simulink model "NPC_MPC_rtiFPGASeparationFile"  (R2018b)
settings: Solver=FixedStepAuto  StartTime=0.0  StopTime=Inf  FixedStep=10e-6  RelTol=1e-3
PostLoadFcn:
  | , if any(exist('dsrtsu_mdlpostloadfcn', 'file') ~= 0), dsrtsu_mdlpostloadfcn('Execute', bdroot); end,
values from neighbouring files (symbols this model uses):
  Amplitude = 1    [params.m]
  L = 10e-3    (= 0.01)    [params.m]
  R = 7.5    [params.m]
  S = [-1 -1 -1 ... (first row only)    [params.m]
undefined symbols (not defined in the file or in its folder): T
libraries: xbsIndex_r4 x282, rti1202lib_adc_class1 x3, rtiproclib x3, simulink x1, rtifpgainterfacelib x1
(part 4 of 6)

== system NPC_MPC_rtiFPGASeparationFile/RTI Data ==
  RTI Data Store : Subsystem  Tag="struct('private',struct('version',struct('dsVer',uint32(2),'dsVerCreation',uint32(2),'RTI',struct('ver','7.13','type','RTI1202')),'access',struct('type','Model','isPerm',1,'created',['24-Mar-2026 14:27:03'],'modified',['24-Mar-2026 17:04:08'],'location','')),'public',struct('main',struct('data',[]),'sub',struct('name',{{'NPC_MPC'}},'data',{{struct('TH',struct('thTaskInfo',struct('taskType',{'TIMER','HWINT','TMRINT','SWINT','GLINT'},'tasksNumOf',{1,1,0,0,0},'srcIds',{{'TIMERA'},{'FPGACL1FPGA_INTP0Ch0'},{},{},{}},'taskNames',{{['Timer Task 1']},{'PROC_INT_BL1'},{},{},{}})),'th_tc',struct('dataType',{'TASK','TASK'},'taskGroupId',{'',''},'taskGroupList',{{},{}},'taskSchedulingPolicy',{'FCFS','FCFS'},'taskType',{'TIMER','HWINT'},'blkh',{-1,['NPC_MPC/PROC_INT_BL1/Common Hardware' char(10) 'Interrupt Interface']},'srcId',{'TIMERA','FPGACL1FPGA_INTP0Ch0'},'srcSgnName',{['Timer A interrupt'],['FPGA Type CL1 FPGA_INT Port 0 Channel 0']},'srcCpuName',{'',''},'taskName',{['Timer Task 1  [1e-05] s'],'PROC_INT_BL1'},'taskNameDisplayExt',{'',''},'smplTime',{1e-5,0},'smplTimeOffs',{0,0},'hasFixedPriority',{0,0},'priority',{1,2},'hasFixedOvc',{0,0},'ovcType',{1,1},'ovcMax',{1,1}),'tc_th',struct('dataType',{'TASK','TASK'},'taskGroupId',{'',''},'taskGroupList',{{},{}},'taskSchedulingPolicy',{'FCFS','FCFS'},'taskType',{'TIMER','HWINT'},'blkh',{-1,['NPC_MPC/PROC_INT_BL1/Common Hardware' char(10) 'Interrupt Interface']},'srcId',{'TIMERA','FPGACL1FPGA_INTP0Ch0'},'srcSgnName',{['Timer A interrupt'],['FPGA Type CL1 FPGA_INT Port 0 Channel 0']},'srcCpuName',{'',''},'taskName',{['Timer Task 1  [1e-05] s'],'PROC_INT_BL1'},'taskNameDisplayExt',{'',''},'smplTime',{1e-5,0},'smplTimeOffs',{0,0},'hasFixedPriority',{0,0},'priority',{1,2},'hasFixedOvc',{0,0},'ovcType',{1,1},'ovcMax',{1,1}))}})))"  mask(RTI_DATA_STORE){}
      mask help:
      | RTI Data Store Block. This block is used by RTI to store internal model dependent data. Deleting this block will result in data loss.
      |
      | NEVER DELETE, COPY, OR MODIFY THIS BLOCK!
      mask Help:
      | RTI Data Store Block. This block is used by RTI to store internal model dependent data. Deleting this block will result in data loss.
      | 
      | NEVER DELETE, COPY, OR MODIFY THIS BLOCK!
      mask Display: text(0.5, 0.5, ' ', 'HorizontalAlignment', 'center');

== system NPC_MPC_rtiFPGASeparationFile/Subsystem ==
  iref : Inport
  i : Inport  Port=2
  Trigger : TriggerPort  TriggerType=function-call  VariantControl=Variant  PortDimensions=1
  Constant : Constant  Value=100
  MATLAB Function : MATLAB Function  TreatAsAtomicUnit=on
  Out1 : Outport
  wires:
  i/1 -> MATLAB Function/2(i)
  MATLAB Function/1(state) -> Out1/1
  iref/1 -> MATLAB Function/1(iref)
  Constant/1 -> MATLAB Function/3(Vdc)

== system NPC_MPC_rtiFPGASeparationFile/FPGA/FPGA_INT_BL1 ==
  Int : Inport
  CEP1 : xbsIndex_r4/Clock Enable Probe  inherit_constraints=off  block_type=ceprobe
      settings: infoedit="Clock enable extractor.  Produces a Boolean output that mirrors the hardware clock enable associated with the input sample rate.<br><br>Hardware notes: in hardware this block costs nothing."
  Constant1 : xbsIndex_r4/Constant  const=1  gui_display_data_type=Fixed-point  arith_type=Boolean  n_bits=16  bin_pt=14  preci_type=Single  exp_width=8  frac_width=24  explicit_period=on  period=1*1e-08  equ=P=C  opselect=C  inp2=PCIN>>17  opr=+  inp1=P  carry=CIN  dbl_ovrd=off  block_type=constant
  Convert1 : xbsIndex_r4/Convert  gui_display_data_type=Fixed-point  arith_type=Unsigned  n_bits=1  bin_pt=0  float_type=Single  exp_bits=8  fraction_bits=24  quantization=Truncate  overflow=Wrap  en=off  latency=0  pipeline=off  dbl_ovrd=off  block_type=convert
  Register1 : xbsIndex_r4/Register  init=0  rst=off  en=on  dbl_ovrd=off  block_type=register
  Terminator : Terminator
  phs_interrupt : Subsystem
  usr_interrupt_00 : xbsIndex_r4/Gateway Out  inherit_from_input=off  hdl_port=on  rows=1  columns=1  UseAsDAC=off  DACChannel='1'  interface=None  automatic_assignment=on  address_offset=hex2dec('00')  intf_name=''  intf_description=''  timing_constraint=None  locs_specified=off  LOCs={}  io_standard={}  block_type=gatewayout
  tag scope: CN_NPC_MPC_1_read_Interrupt_1_data_o=global
  wires:
  phs_interrupt/1(data_o) -> [CN_NPC_MPC_1_read_Interrupt_1_data_o], Terminator/1
  usr_interrupt_00/1 -> phs_interrupt/1(data_i)
  Convert1/1 -> Register1/1
  Int/1 -> Convert1/1
  Register1/1 -> usr_interrupt_00/1
  CEP1/1 -> Register1/2
  Constant1/1 -> CEP1/1

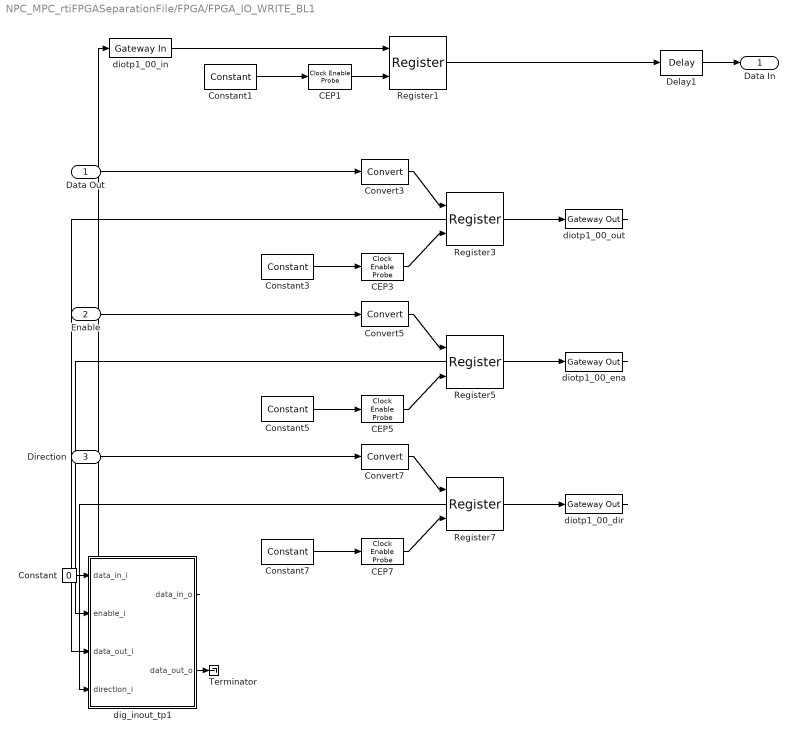
== system NPC_MPC_rtiFPGASeparationFile/FPGA/FPGA_IO_WRITE_BL1 ==
  Data Out : Inport
  Enable : Inport  Port=2
  Direction : Inport  Port=3
  CEP{1,3,5,7} (4 alike) : xbsIndex_r4/Clock Enable Probe  inherit_constraints=off  block_type=ceprobe
      settings: infoedit="Clock enable extractor.  Produces a Boolean output that mirrors the hardware clock enable associated with the input sample rate.<br><br>Hardware notes: in hardware this block costs nothing."
  Constant : Constant  Value=0
  Constant{1,3,5,7} (4 alike) : xbsIndex_r4/Constant  const=1  gui_display_data_type=Fixed-point  arith_type=Boolean  n_bits=16  bin_pt=14  preci_type=Single  exp_width=8  frac_width=24  explicit_period=on  period=1*1e-08  equ=P=C  opselect=C  inp2=PCIN>>17  opr=+  inp1=P  carry=CIN  dbl_ovrd=off  block_type=constant
  Convert3 : xbsIndex_r4/Convert  gui_display_data_type=Fixed-point  arith_type=Unsigned  n_bits=1  bin_pt=0  float_type=Single  exp_bits=8  fraction_bits=24  quantization=Truncate  overflow=Wrap  en=off  latency=0  pipeline=off  dbl_ovrd=off  block_type=convert
  Convert5 : xbsIndex_r4/Convert  gui_display_data_type=Fixed-point  arith_type=Unsigned  n_bits=1  bin_pt=0  float_type=Single  exp_bits=8  fraction_bits=24  quantization=Truncate  overflow=Wrap  en=off  latency=0  pipeline=off  dbl_ovrd=off  block_type=convert
  Convert7 : xbsIndex_r4/Convert  gui_display_data_type=Fixed-point  arith_type=Unsigned  n_bits=1  bin_pt=0  float_type=Single  exp_bits=8  fraction_bits=24  quantization=Truncate  overflow=Wrap  en=off  latency=0  pipeline=off  dbl_ovrd=off  block_type=convert
  Delay1 : xbsIndex_r4/Delay  rst=off  infoeditControl=Selection of Reset will increase slice count due to use of real FFs and instead of SRLs  en=off  latency=0  reg_retiming=off  dbl_ovrd=off  block_type=delay
  Register{1,3,5,7} (4 alike) : xbsIndex_r4/Register  init=0  rst=off  en=on  dbl_ovrd=off  block_type=register
  Terminator : Terminator
  dig_inout_tp1 : Subsystem
      mask init:
      | par = rtifpgafcnlib('GetCurrentParaValue', get_param(get(gcbh, 'parent'), 'handle'));
      | inverted_dio = str2double(par(2).Value{1});
      | vsetting = str2double(par(5).Value{1});
      | switch vsetting 
      |     case 1
      |         voltage = 3.3
      |     case 2
      |         voltage = 2.5;
      |     otherwise
      |         voltage = 5;
      | end
  diotp1_00_dir : xbsIndex_r4/Gateway Out  inherit_from_input=off  hdl_port=on  rows=1  columns=1  UseAsDAC=off  DACChannel='1'  interface=None  automatic_assignment=on  address_offset=hex2dec('00')  intf_name=''  intf_description=''  timing_constraint=None  locs_specified=off  LOCs={}  io_standard={}  block_type=gatewayout
  diotp1_00_ena : xbsIndex_r4/Gateway Out  inherit_from_input=off  hdl_port=on  rows=1  columns=1  UseAsDAC=off  DACChannel='1'  interface=None  automatic_assignment=on  address_offset=hex2dec('00')  intf_name=''  intf_description=''  timing_constraint=None  locs_specified=off  LOCs={}  io_standard={}  block_type=gatewayout
  diotp1_00_in : xbsIndex_r4/Gateway In  gui_display_data_type=Fixed-point  arith_type=Unsigned  n_bits=1  bin_pt=0  preci_type=Single  exp_width=8  frac_width=24  rows=1  columns=1  quantization="Round  (unbiased: +/- Inf)"  overflow=Saturate  period=1e-08  UseAsADC=off  ADCChannel='1'  interface=None  automatic_assignment=on  address_offset=hex2dec('00')  intf_name=''  intf_description=''  default_value=0  timing_constraint=None  locs_specified=off  LOCs={}  io_standard={}  inherit_from_input=off  hdl_port=on  dbl_ovrd=off  block_type=gatewayin
  diotp1_00_out : xbsIndex_r4/Gateway Out  inherit_from_input=off  hdl_port=on  rows=1  columns=1  UseAsDAC=off  DACChannel='1'  interface=None  automatic_assignment=on  address_offset=hex2dec('00')  intf_name=''  intf_description=''  timing_constraint=None  locs_specified=off  LOCs={}  io_standard={}  block_type=gatewayout
  Data In : Outport
  wires:
  dig_inout_tp1/2(data_out_o) -> Terminator/1
  Constant/1 -> dig_inout_tp1/1(data_in_i)
  diotp1_00_dir/1 -> dig_inout_tp1/4(direction_i)
  diotp1_00_ena/1 -> dig_inout_tp1/2(enable_i)
  diotp1_00_out/1 -> dig_inout_tp1/3(data_out_i)
  dig_inout_tp1/1(data_in_o) -> diotp1_00_in/1
  Convert7/1 -> Register7/1
  Direction/1 -> Convert7/1
  Register7/1 -> diotp1_00_dir/1
  CEP7/1 -> Register7/2
  Constant7/1 -> CEP7/1
  Convert5/1 -> Register5/1
  Enable/1 -> Convert5/1
  Register5/1 -> diotp1_00_ena/1
  CEP5/1 -> Register5/2
  Constant5/1 -> CEP5/1
  Convert3/1 -> Register3/1
  Data Out/1 -> Convert3/1
  Register3/1 -> diotp1_00_out/1
  CEP3/1 -> Register3/2
  Constant3/1 -> CEP3/1
  diotp1_00_in/1 -> Register1/1
  CEP1/1 -> Register1/2
  Constant1/1 -> CEP1/1
  Delay1/1 -> Data In/1
  Register1/1 -> Delay1/1

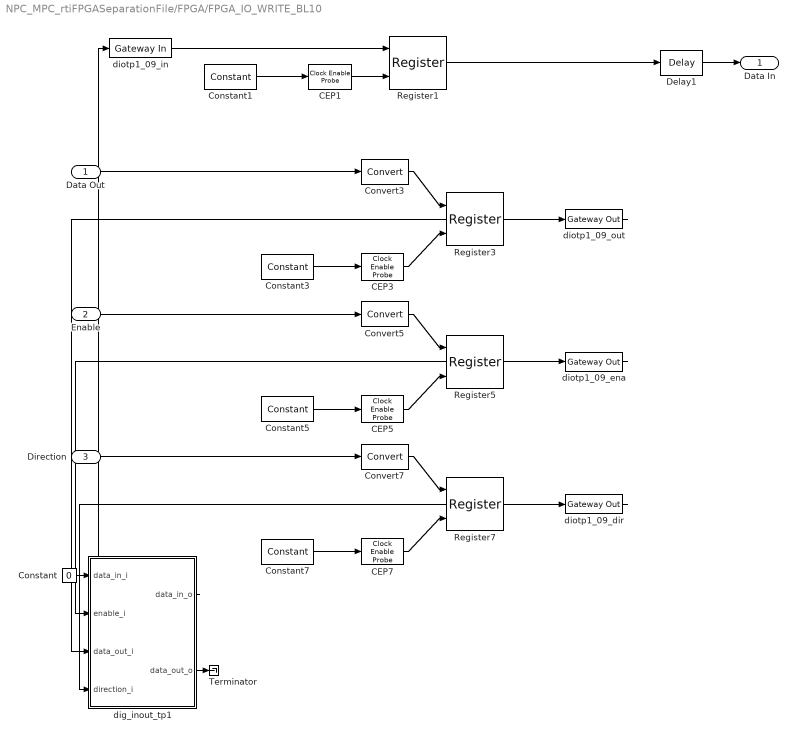
== system NPC_MPC_rtiFPGASeparationFile/FPGA/FPGA_IO_WRITE_BL10 ==
  Data Out : Inport
  Enable : Inport  Port=2
  Direction : Inport  Port=3
  CEP{1,3,5,7} (4 alike) : xbsIndex_r4/Clock Enable Probe  inherit_constraints=off  block_type=ceprobe
      settings: infoedit="Clock enable extractor.  Produces a Boolean output that mirrors the hardware clock enable associated with the input sample rate.<br><br>Hardware notes: in hardware this block costs nothing."
  Constant : Constant  Value=0
  Constant{1,3,5,7} (4 alike) : xbsIndex_r4/Constant  const=1  gui_display_data_type=Fixed-point  arith_type=Boolean  n_bits=16  bin_pt=14  preci_type=Single  exp_width=8  frac_width=24  explicit_period=on  period=1*1e-08  equ=P=C  opselect=C  inp2=PCIN>>17  opr=+  inp1=P  carry=CIN  dbl_ovrd=off  block_type=constant
  Convert3 : xbsIndex_r4/Convert  gui_display_data_type=Fixed-point  arith_type=Unsigned  n_bits=1  bin_pt=0  float_type=Single  exp_bits=8  fraction_bits=24  quantization=Truncate  overflow=Wrap  en=off  latency=0  pipeline=off  dbl_ovrd=off  block_type=convert
  Convert5 : xbsIndex_r4/Convert  gui_display_data_type=Fixed-point  arith_type=Unsigned  n_bits=1  bin_pt=0  float_type=Single  exp_bits=8  fraction_bits=24  quantization=Truncate  overflow=Wrap  en=off  latency=0  pipeline=off  dbl_ovrd=off  block_type=convert
  Convert7 : xbsIndex_r4/Convert  gui_display_data_type=Fixed-point  arith_type=Unsigned  n_bits=1  bin_pt=0  float_type=Single  exp_bits=8  fraction_bits=24  quantization=Truncate  overflow=Wrap  en=off  latency=0  pipeline=off  dbl_ovrd=off  block_type=convert
  Delay1 : xbsIndex_r4/Delay  rst=off  infoeditControl=Selection of Reset will increase slice count due to use of real FFs and instead of SRLs  en=off  latency=0  reg_retiming=off  dbl_ovrd=off  block_type=delay
  Register{1,3,5,7} (4 alike) : xbsIndex_r4/Register  init=0  rst=off  en=on  dbl_ovrd=off  block_type=register
  Terminator : Terminator
  dig_inout_tp1 : Subsystem
      mask init: same as NPC_MPC_rtiFPGASeparationFile/FPGA/FPGA_IO_WRITE_BL1/dig_inout_tp1
  diotp1_09_dir : xbsIndex_r4/Gateway Out  inherit_from_input=off  hdl_port=on  rows=1  columns=1  UseAsDAC=off  DACChannel='1'  interface=None  automatic_assignment=on  address_offset=hex2dec('00')  intf_name=''  intf_description=''  timing_constraint=None  locs_specified=off  LOCs={}  io_standard={}  block_type=gatewayout
  diotp1_09_ena : xbsIndex_r4/Gateway Out  inherit_from_input=off  hdl_port=on  rows=1  columns=1  UseAsDAC=off  DACChannel='1'  interface=None  automatic_assignment=on  address_offset=hex2dec('00')  intf_name=''  intf_description=''  timing_constraint=None  locs_specified=off  LOCs={}  io_standard={}  block_type=gatewayout
  diotp1_09_in : xbsIndex_r4/Gateway In  gui_display_data_type=Fixed-point  arith_type=Unsigned  n_bits=1  bin_pt=0  preci_type=Single  exp_width=8  frac_width=24  rows=1  columns=1  quantization="Round  (unbiased: +/- Inf)"  overflow=Saturate  period=1e-08  UseAsADC=off  ADCChannel='1'  interface=None  automatic_assignment=on  address_offset=hex2dec('00')  intf_name=''  intf_description=''  default_value=0  timing_constraint=None  locs_specified=off  LOCs={}  io_standard={}  inherit_from_input=off  hdl_port=on  dbl_ovrd=off  block_type=gatewayin
  diotp1_09_out : xbsIndex_r4/Gateway Out  inherit_from_input=off  hdl_port=on  rows=1  columns=1  UseAsDAC=off  DACChannel='1'  interface=None  automatic_assignment=on  address_offset=hex2dec('00')  intf_name=''  intf_description=''  timing_constraint=None  locs_specified=off  LOCs={}  io_standard={}  block_type=gatewayout
  Data In : Outport
  wires:
  dig_inout_tp1/2(data_out_o) -> Terminator/1
  Constant/1 -> dig_inout_tp1/1(data_in_i)
  diotp1_09_dir/1 -> dig_inout_tp1/4(direction_i)
  diotp1_09_ena/1 -> dig_inout_tp1/2(enable_i)
  diotp1_09_out/1 -> dig_inout_tp1/3(data_out_i)
  dig_inout_tp1/1(data_in_o) -> diotp1_09_in/1
  Convert7/1 -> Register7/1
  Direction/1 -> Convert7/1
  Register7/1 -> diotp1_09_dir/1
  CEP7/1 -> Register7/2
  Constant7/1 -> CEP7/1
  Convert5/1 -> Register5/1
  Enable/1 -> Convert5/1
  Register5/1 -> diotp1_09_ena/1
  CEP5/1 -> Register5/2
  Constant5/1 -> CEP5/1
  Convert3/1 -> Register3/1
  Data Out/1 -> Convert3/1
  Register3/1 -> diotp1_09_out/1
  CEP3/1 -> Register3/2
  Constant3/1 -> CEP3/1
  diotp1_09_in/1 -> Register1/1
  CEP1/1 -> Register1/2
  Constant1/1 -> CEP1/1
  Delay1/1 -> Data In/1
  Register1/1 -> Delay1/1

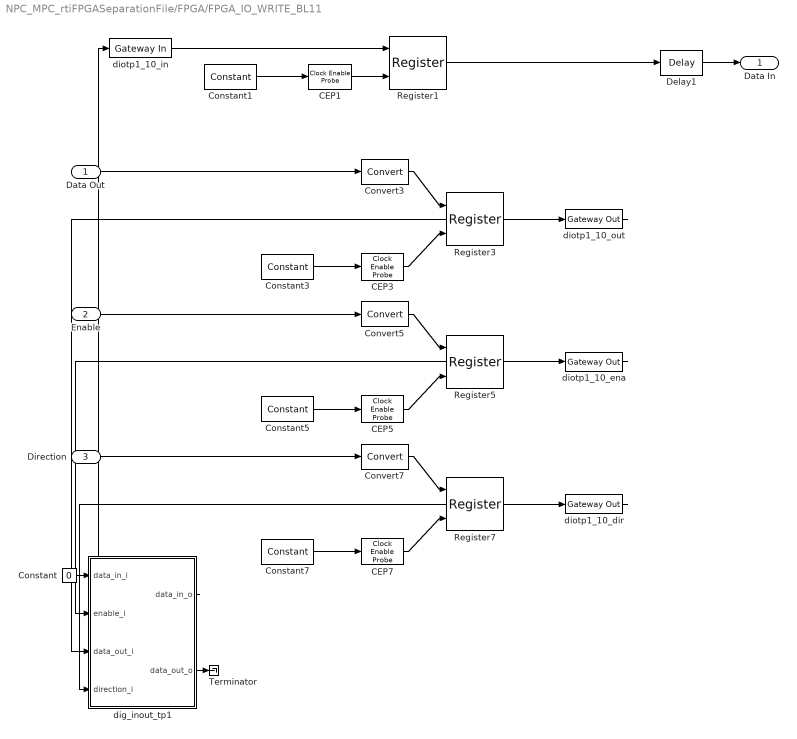
== system NPC_MPC_rtiFPGASeparationFile/FPGA/FPGA_IO_WRITE_BL11 ==
  Data Out : Inport
  Enable : Inport  Port=2
  Direction : Inport  Port=3
  CEP{1,3,5,7} (4 alike) : xbsIndex_r4/Clock Enable Probe  inherit_constraints=off  block_type=ceprobe
      settings: infoedit="Clock enable extractor.  Produces a Boolean output that mirrors the hardware clock enable associated with the input sample rate.<br><br>Hardware notes: in hardware this block costs nothing."
  Constant : Constant  Value=0
  Constant{1,3,5,7} (4 alike) : xbsIndex_r4/Constant  const=1  gui_display_data_type=Fixed-point  arith_type=Boolean  n_bits=16  bin_pt=14  preci_type=Single  exp_width=8  frac_width=24  explicit_period=on  period=1*1e-08  equ=P=C  opselect=C  inp2=PCIN>>17  opr=+  inp1=P  carry=CIN  dbl_ovrd=off  block_type=constant
  Convert3 : xbsIndex_r4/Convert  gui_display_data_type=Fixed-point  arith_type=Unsigned  n_bits=1  bin_pt=0  float_type=Single  exp_bits=8  fraction_bits=24  quantization=Truncate  overflow=Wrap  en=off  latency=0  pipeline=off  dbl_ovrd=off  block_type=convert
  Convert5 : xbsIndex_r4/Convert  gui_display_data_type=Fixed-point  arith_type=Unsigned  n_bits=1  bin_pt=0  float_type=Single  exp_bits=8  fraction_bits=24  quantization=Truncate  overflow=Wrap  en=off  latency=0  pipeline=off  dbl_ovrd=off  block_type=convert
  Convert7 : xbsIndex_r4/Convert  gui_display_data_type=Fixed-point  arith_type=Unsigned  n_bits=1  bin_pt=0  float_type=Single  exp_bits=8  fraction_bits=24  quantization=Truncate  overflow=Wrap  en=off  latency=0  pipeline=off  dbl_ovrd=off  block_type=convert
  Delay1 : xbsIndex_r4/Delay  rst=off  infoeditControl=Selection of Reset will increase slice count due to use of real FFs and instead of SRLs  en=off  latency=0  reg_retiming=off  dbl_ovrd=off  block_type=delay
  Register{1,3,5,7} (4 alike) : xbsIndex_r4/Register  init=0  rst=off  en=on  dbl_ovrd=off  block_type=register
  Terminator : Terminator
  dig_inout_tp1 : Subsystem
      mask init: same as NPC_MPC_rtiFPGASeparationFile/FPGA/FPGA_IO_WRITE_BL1/dig_inout_tp1
  diotp1_10_dir : xbsIndex_r4/Gateway Out  inherit_from_input=off  hdl_port=on  rows=1  columns=1  UseAsDAC=off  DACChannel='1'  interface=None  automatic_assignment=on  address_offset=hex2dec('00')  intf_name=''  intf_description=''  timing_constraint=None  locs_specified=off  LOCs={}  io_standard={}  block_type=gatewayout
  diotp1_10_ena : xbsIndex_r4/Gateway Out  inherit_from_input=off  hdl_port=on  rows=1  columns=1  UseAsDAC=off  DACChannel='1'  interface=None  automatic_assignment=on  address_offset=hex2dec('00')  intf_name=''  intf_description=''  timing_constraint=None  locs_specified=off  LOCs={}  io_standard={}  block_type=gatewayout
  diotp1_10_in : xbsIndex_r4/Gateway In  gui_display_data_type=Fixed-point  arith_type=Unsigned  n_bits=1  bin_pt=0  preci_type=Single  exp_width=8  frac_width=24  rows=1  columns=1  quantization="Round  (unbiased: +/- Inf)"  overflow=Saturate  period=1e-08  UseAsADC=off  ADCChannel='1'  interface=None  automatic_assignment=on  address_offset=hex2dec('00')  intf_name=''  intf_description=''  default_value=0  timing_constraint=None  locs_specified=off  LOCs={}  io_standard={}  inherit_from_input=off  hdl_port=on  dbl_ovrd=off  block_type=gatewayin
  diotp1_10_out : xbsIndex_r4/Gateway Out  inherit_from_input=off  hdl_port=on  rows=1  columns=1  UseAsDAC=off  DACChannel='1'  interface=None  automatic_assignment=on  address_offset=hex2dec('00')  intf_name=''  intf_description=''  timing_constraint=None  locs_specified=off  LOCs={}  io_standard={}  block_type=gatewayout
  Data In : Outport
  wires:
  dig_inout_tp1/2(data_out_o) -> Terminator/1
  Constant/1 -> dig_inout_tp1/1(data_in_i)
  diotp1_10_dir/1 -> dig_inout_tp1/4(direction_i)
  diotp1_10_ena/1 -> dig_inout_tp1/2(enable_i)
  diotp1_10_out/1 -> dig_inout_tp1/3(data_out_i)
  dig_inout_tp1/1(data_in_o) -> diotp1_10_in/1
  Convert7/1 -> Register7/1
  Direction/1 -> Convert7/1
  Register7/1 -> diotp1_10_dir/1
  CEP7/1 -> Register7/2
  Constant7/1 -> CEP7/1
  Convert5/1 -> Register5/1
  Enable/1 -> Convert5/1
  Register5/1 -> diotp1_10_ena/1
  CEP5/1 -> Register5/2
  Constant5/1 -> CEP5/1
  Convert3/1 -> Register3/1
  Data Out/1 -> Convert3/1
  Register3/1 -> diotp1_10_out/1
  CEP3/1 -> Register3/2
  Constant3/1 -> CEP3/1
  diotp1_10_in/1 -> Register1/1
  CEP1/1 -> Register1/2
  Constant1/1 -> CEP1/1
  Delay1/1 -> Data In/1
  Register1/1 -> Delay1/1

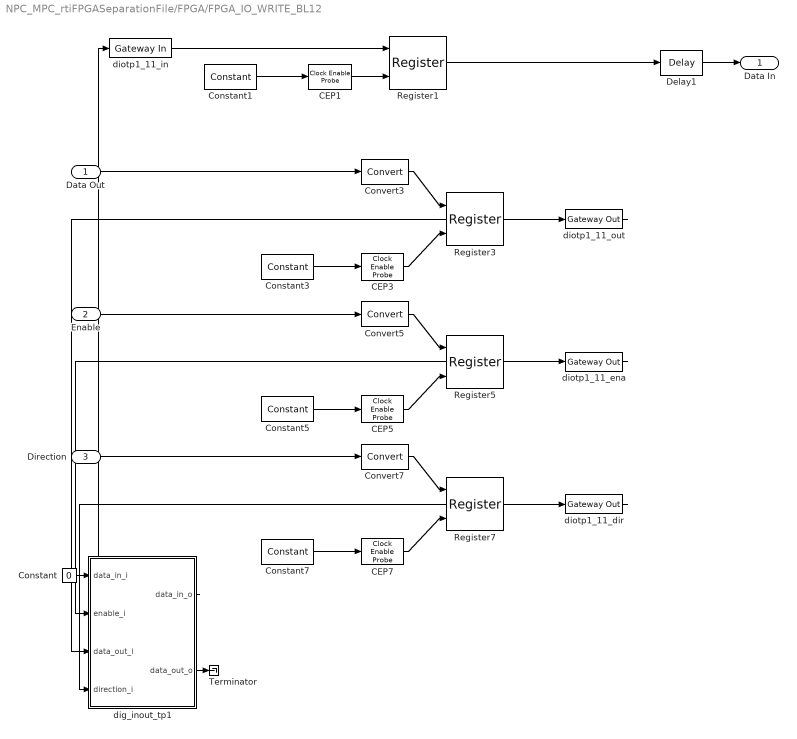
== system NPC_MPC_rtiFPGASeparationFile/FPGA/FPGA_IO_WRITE_BL12 ==
  Data Out : Inport
  Enable : Inport  Port=2
  Direction : Inport  Port=3
  CEP{1,3,5,7} (4 alike) : xbsIndex_r4/Clock Enable Probe  inherit_constraints=off  block_type=ceprobe
      settings: infoedit="Clock enable extractor.  Produces a Boolean output that mirrors the hardware clock enable associated with the input sample rate.<br><br>Hardware notes: in hardware this block costs nothing."
  Constant : Constant  Value=0
  Constant{1,3,5,7} (4 alike) : xbsIndex_r4/Constant  const=1  gui_display_data_type=Fixed-point  arith_type=Boolean  n_bits=16  bin_pt=14  preci_type=Single  exp_width=8  frac_width=24  explicit_period=on  period=1*1e-08  equ=P=C  opselect=C  inp2=PCIN>>17  opr=+  inp1=P  carry=CIN  dbl_ovrd=off  block_type=constant
  Convert3 : xbsIndex_r4/Convert  gui_display_data_type=Fixed-point  arith_type=Unsigned  n_bits=1  bin_pt=0  float_type=Single  exp_bits=8  fraction_bits=24  quantization=Truncate  overflow=Wrap  en=off  latency=0  pipeline=off  dbl_ovrd=off  block_type=convert
  Convert5 : xbsIndex_r4/Convert  gui_display_data_type=Fixed-point  arith_type=Unsigned  n_bits=1  bin_pt=0  float_type=Single  exp_bits=8  fraction_bits=24  quantization=Truncate  overflow=Wrap  en=off  latency=0  pipeline=off  dbl_ovrd=off  block_type=convert
  Convert7 : xbsIndex_r4/Convert  gui_display_data_type=Fixed-point  arith_type=Unsigned  n_bits=1  bin_pt=0  float_type=Single  exp_bits=8  fraction_bits=24  quantization=Truncate  overflow=Wrap  en=off  latency=0  pipeline=off  dbl_ovrd=off  block_type=convert
  Delay1 : xbsIndex_r4/Delay  rst=off  infoeditControl=Selection of Reset will increase slice count due to use of real FFs and instead of SRLs  en=off  latency=0  reg_retiming=off  dbl_ovrd=off  block_type=delay
  Register{1,3,5,7} (4 alike) : xbsIndex_r4/Register  init=0  rst=off  en=on  dbl_ovrd=off  block_type=register
  Terminator : Terminator
  dig_inout_tp1 : Subsystem
      mask init: same as NPC_MPC_rtiFPGASeparationFile/FPGA/FPGA_IO_WRITE_BL1/dig_inout_tp1
  diotp1_11_dir : xbsIndex_r4/Gateway Out  inherit_from_input=off  hdl_port=on  rows=1  columns=1  UseAsDAC=off  DACChannel='1'  interface=None  automatic_assignment=on  address_offset=hex2dec('00')  intf_name=''  intf_description=''  timing_constraint=None  locs_specified=off  LOCs={}  io_standard={}  block_type=gatewayout
  diotp1_11_ena : xbsIndex_r4/Gateway Out  inherit_from_input=off  hdl_port=on  rows=1  columns=1  UseAsDAC=off  DACChannel='1'  interface=None  automatic_assignment=on  address_offset=hex2dec('00')  intf_name=''  intf_description=''  timing_constraint=None  locs_specified=off  LOCs={}  io_standard={}  block_type=gatewayout
  diotp1_11_in : xbsIndex_r4/Gateway In  gui_display_data_type=Fixed-point  arith_type=Unsigned  n_bits=1  bin_pt=0  preci_type=Single  exp_width=8  frac_width=24  rows=1  columns=1  quantization="Round  (unbiased: +/- Inf)"  overflow=Saturate  period=1e-08  UseAsADC=off  ADCChannel='1'  interface=None  automatic_assignment=on  address_offset=hex2dec('00')  intf_name=''  intf_description=''  default_value=0  timing_constraint=None  locs_specified=off  LOCs={}  io_standard={}  inherit_from_input=off  hdl_port=on  dbl_ovrd=off  block_type=gatewayin
  diotp1_11_out : xbsIndex_r4/Gateway Out  inherit_from_input=off  hdl_port=on  rows=1  columns=1  UseAsDAC=off  DACChannel='1'  interface=None  automatic_assignment=on  address_offset=hex2dec('00')  intf_name=''  intf_description=''  timing_constraint=None  locs_specified=off  LOCs={}  io_standard={}  block_type=gatewayout
  Data In : Outport
  wires:
  dig_inout_tp1/2(data_out_o) -> Terminator/1
  Constant/1 -> dig_inout_tp1/1(data_in_i)
  diotp1_11_dir/1 -> dig_inout_tp1/4(direction_i)
  diotp1_11_ena/1 -> dig_inout_tp1/2(enable_i)
  diotp1_11_out/1 -> dig_inout_tp1/3(data_out_i)
  dig_inout_tp1/1(data_in_o) -> diotp1_11_in/1
  Convert7/1 -> Register7/1
  Direction/1 -> Convert7/1
  Register7/1 -> diotp1_11_dir/1
  CEP7/1 -> Register7/2
  Constant7/1 -> CEP7/1
  Convert5/1 -> Register5/1
  Enable/1 -> Convert5/1
  Register5/1 -> diotp1_11_ena/1
  CEP5/1 -> Register5/2
  Constant5/1 -> CEP5/1
  Convert3/1 -> Register3/1
  Data Out/1 -> Convert3/1
  Register3/1 -> diotp1_11_out/1
  CEP3/1 -> Register3/2
  Constant3/1 -> CEP3/1
  diotp1_11_in/1 -> Register1/1
  CEP1/1 -> Register1/2
  Constant1/1 -> CEP1/1
  Delay1/1 -> Data In/1
  Register1/1 -> Delay1/1

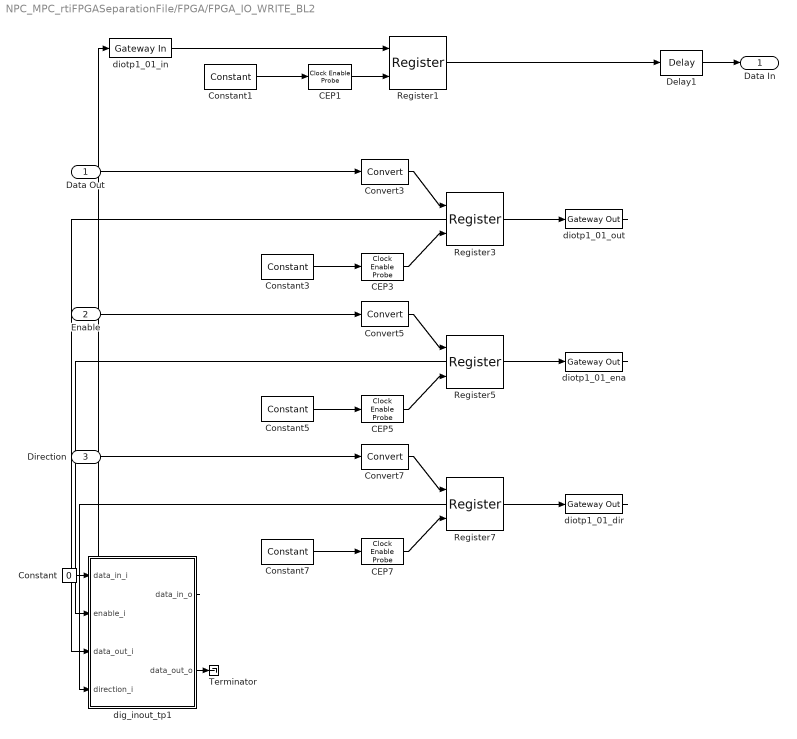
== system NPC_MPC_rtiFPGASeparationFile/FPGA/FPGA_IO_WRITE_BL2 ==
  Data Out : Inport
  Enable : Inport  Port=2
  Direction : Inport  Port=3
  CEP{1,3,5,7} (4 alike) : xbsIndex_r4/Clock Enable Probe  inherit_constraints=off  block_type=ceprobe
      settings: infoedit="Clock enable extractor.  Produces a Boolean output that mirrors the hardware clock enable associated with the input sample rate.<br><br>Hardware notes: in hardware this block costs nothing."
  Constant : Constant  Value=0
  Constant{1,3,5,7} (4 alike) : xbsIndex_r4/Constant  const=1  gui_display_data_type=Fixed-point  arith_type=Boolean  n_bits=16  bin_pt=14  preci_type=Single  exp_width=8  frac_width=24  explicit_period=on  period=1*1e-08  equ=P=C  opselect=C  inp2=PCIN>>17  opr=+  inp1=P  carry=CIN  dbl_ovrd=off  block_type=constant
  Convert3 : xbsIndex_r4/Convert  gui_display_data_type=Fixed-point  arith_type=Unsigned  n_bits=1  bin_pt=0  float_type=Single  exp_bits=8  fraction_bits=24  quantization=Truncate  overflow=Wrap  en=off  latency=0  pipeline=off  dbl_ovrd=off  block_type=convert
  Convert5 : xbsIndex_r4/Convert  gui_display_data_type=Fixed-point  arith_type=Unsigned  n_bits=1  bin_pt=0  float_type=Single  exp_bits=8  fraction_bits=24  quantization=Truncate  overflow=Wrap  en=off  latency=0  pipeline=off  dbl_ovrd=off  block_type=convert
  Convert7 : xbsIndex_r4/Convert  gui_display_data_type=Fixed-point  arith_type=Unsigned  n_bits=1  bin_pt=0  float_type=Single  exp_bits=8  fraction_bits=24  quantization=Truncate  overflow=Wrap  en=off  latency=0  pipeline=off  dbl_ovrd=off  block_type=convert
  Delay1 : xbsIndex_r4/Delay  rst=off  infoeditControl=Selection of Reset will increase slice count due to use of real FFs and instead of SRLs  en=off  latency=0  reg_retiming=off  dbl_ovrd=off  block_type=delay
  Register{1,3,5,7} (4 alike) : xbsIndex_r4/Register  init=0  rst=off  en=on  dbl_ovrd=off  block_type=register
  Terminator : Terminator
  dig_inout_tp1 : Subsystem
      mask init: same as NPC_MPC_rtiFPGASeparationFile/FPGA/FPGA_IO_WRITE_BL1/dig_inout_tp1
  diotp1_01_dir : xbsIndex_r4/Gateway Out  inherit_from_input=off  hdl_port=on  rows=1  columns=1  UseAsDAC=off  DACChannel='1'  interface=None  automatic_assignment=on  address_offset=hex2dec('00')  intf_name=''  intf_description=''  timing_constraint=None  locs_specified=off  LOCs={}  io_standard={}  block_type=gatewayout
  diotp1_01_ena : xbsIndex_r4/Gateway Out  inherit_from_input=off  hdl_port=on  rows=1  columns=1  UseAsDAC=off  DACChannel='1'  interface=None  automatic_assignment=on  address_offset=hex2dec('00')  intf_name=''  intf_description=''  timing_constraint=None  locs_specified=off  LOCs={}  io_standard={}  block_type=gatewayout
  diotp1_01_in : xbsIndex_r4/Gateway In  gui_display_data_type=Fixed-point  arith_type=Unsigned  n_bits=1  bin_pt=0  preci_type=Single  exp_width=8  frac_width=24  rows=1  columns=1  quantization="Round  (unbiased: +/- Inf)"  overflow=Saturate  period=1e-08  UseAsADC=off  ADCChannel='1'  interface=None  automatic_assignment=on  address_offset=hex2dec('00')  intf_name=''  intf_description=''  default_value=0  timing_constraint=None  locs_specified=off  LOCs={}  io_standard={}  inherit_from_input=off  hdl_port=on  dbl_ovrd=off  block_type=gatewayin
  diotp1_01_out : xbsIndex_r4/Gateway Out  inherit_from_input=off  hdl_port=on  rows=1  columns=1  UseAsDAC=off  DACChannel='1'  interface=None  automatic_assignment=on  address_offset=hex2dec('00')  intf_name=''  intf_description=''  timing_constraint=None  locs_specified=off  LOCs={}  io_standard={}  block_type=gatewayout
  Data In : Outport
  wires:
  dig_inout_tp1/2(data_out_o) -> Terminator/1
  Constant/1 -> dig_inout_tp1/1(data_in_i)
  diotp1_01_dir/1 -> dig_inout_tp1/4(direction_i)
  diotp1_01_ena/1 -> dig_inout_tp1/2(enable_i)
  diotp1_01_out/1 -> dig_inout_tp1/3(data_out_i)
  dig_inout_tp1/1(data_in_o) -> diotp1_01_in/1
  Convert7/1 -> Register7/1
  Direction/1 -> Convert7/1
  Register7/1 -> diotp1_01_dir/1
  CEP7/1 -> Register7/2
  Constant7/1 -> CEP7/1
  Convert5/1 -> Register5/1
  Enable/1 -> Convert5/1
  Register5/1 -> diotp1_01_ena/1
  CEP5/1 -> Register5/2
  Constant5/1 -> CEP5/1
  Convert3/1 -> Register3/1
  Data Out/1 -> Convert3/1
  Register3/1 -> diotp1_01_out/1
  CEP3/1 -> Register3/2
  Constant3/1 -> CEP3/1
  diotp1_01_in/1 -> Register1/1
  CEP1/1 -> Register1/2
  Constant1/1 -> CEP1/1
  Delay1/1 -> Data In/1
  Register1/1 -> Delay1/1

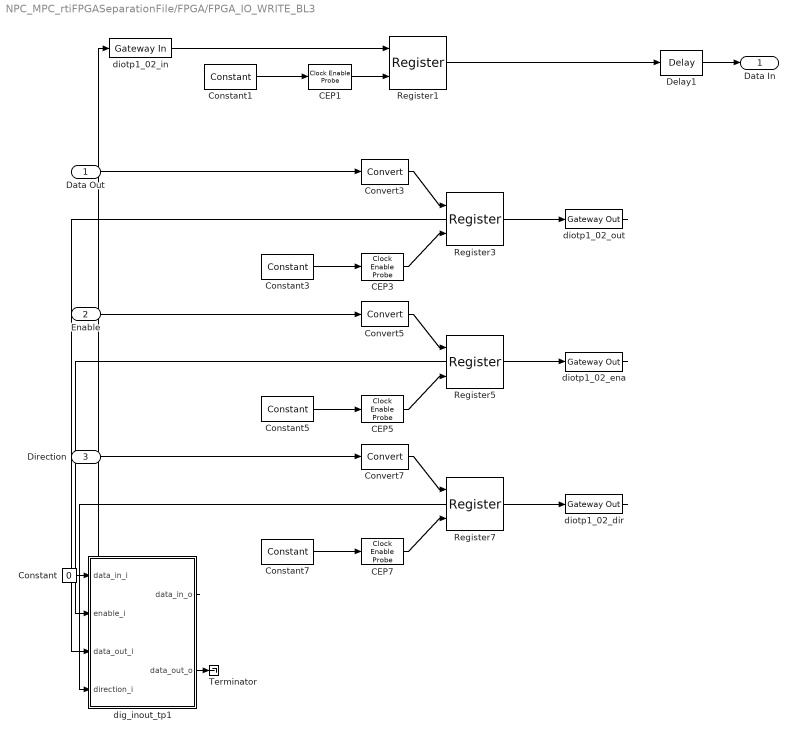
== system NPC_MPC_rtiFPGASeparationFile/FPGA/FPGA_IO_WRITE_BL3 ==
  Data Out : Inport
  Enable : Inport  Port=2
  Direction : Inport  Port=3
  CEP{1,3,5,7} (4 alike) : xbsIndex_r4/Clock Enable Probe  inherit_constraints=off  block_type=ceprobe
      settings: infoedit="Clock enable extractor.  Produces a Boolean output that mirrors the hardware clock enable associated with the input sample rate.<br><br>Hardware notes: in hardware this block costs nothing."
  Constant : Constant  Value=0
  Constant{1,3,5,7} (4 alike) : xbsIndex_r4/Constant  const=1  gui_display_data_type=Fixed-point  arith_type=Boolean  n_bits=16  bin_pt=14  preci_type=Single  exp_width=8  frac_width=24  explicit_period=on  period=1*1e-08  equ=P=C  opselect=C  inp2=PCIN>>17  opr=+  inp1=P  carry=CIN  dbl_ovrd=off  block_type=constant
  Convert3 : xbsIndex_r4/Convert  gui_display_data_type=Fixed-point  arith_type=Unsigned  n_bits=1  bin_pt=0  float_type=Single  exp_bits=8  fraction_bits=24  quantization=Truncate  overflow=Wrap  en=off  latency=0  pipeline=off  dbl_ovrd=off  block_type=convert
  Convert5 : xbsIndex_r4/Convert  gui_display_data_type=Fixed-point  arith_type=Unsigned  n_bits=1  bin_pt=0  float_type=Single  exp_bits=8  fraction_bits=24  quantization=Truncate  overflow=Wrap  en=off  latency=0  pipeline=off  dbl_ovrd=off  block_type=convert
  Convert7 : xbsIndex_r4/Convert  gui_display_data_type=Fixed-point  arith_type=Unsigned  n_bits=1  bin_pt=0  float_type=Single  exp_bits=8  fraction_bits=24  quantization=Truncate  overflow=Wrap  en=off  latency=0  pipeline=off  dbl_ovrd=off  block_type=convert
  Delay1 : xbsIndex_r4/Delay  rst=off  infoeditControl=Selection of Reset will increase slice count due to use of real FFs and instead of SRLs  en=off  latency=0  reg_retiming=off  dbl_ovrd=off  block_type=delay
  Register{1,3,5,7} (4 alike) : xbsIndex_r4/Register  init=0  rst=off  en=on  dbl_ovrd=off  block_type=register
  Terminator : Terminator
  dig_inout_tp1 : Subsystem
      mask init: same as NPC_MPC_rtiFPGASeparationFile/FPGA/FPGA_IO_WRITE_BL1/dig_inout_tp1
  diotp1_02_dir : xbsIndex_r4/Gateway Out  inherit_from_input=off  hdl_port=on  rows=1  columns=1  UseAsDAC=off  DACChannel='1'  interface=None  automatic_assignment=on  address_offset=hex2dec('00')  intf_name=''  intf_description=''  timing_constraint=None  locs_specified=off  LOCs={}  io_standard={}  block_type=gatewayout
  diotp1_02_ena : xbsIndex_r4/Gateway Out  inherit_from_input=off  hdl_port=on  rows=1  columns=1  UseAsDAC=off  DACChannel='1'  interface=None  automatic_assignment=on  address_offset=hex2dec('00')  intf_name=''  intf_description=''  timing_constraint=None  locs_specified=off  LOCs={}  io_standard={}  block_type=gatewayout
  diotp1_02_in : xbsIndex_r4/Gateway In  gui_display_data_type=Fixed-point  arith_type=Unsigned  n_bits=1  bin_pt=0  preci_type=Single  exp_width=8  frac_width=24  rows=1  columns=1  quantization="Round  (unbiased: +/- Inf)"  overflow=Saturate  period=1e-08  UseAsADC=off  ADCChannel='1'  interface=None  automatic_assignment=on  address_offset=hex2dec('00')  intf_name=''  intf_description=''  default_value=0  timing_constraint=None  locs_specified=off  LOCs={}  io_standard={}  inherit_from_input=off  hdl_port=on  dbl_ovrd=off  block_type=gatewayin
  diotp1_02_out : xbsIndex_r4/Gateway Out  inherit_from_input=off  hdl_port=on  rows=1  columns=1  UseAsDAC=off  DACChannel='1'  interface=None  automatic_assignment=on  address_offset=hex2dec('00')  intf_name=''  intf_description=''  timing_constraint=None  locs_specified=off  LOCs={}  io_standard={}  block_type=gatewayout
  Data In : Outport
  wires:
  dig_inout_tp1/2(data_out_o) -> Terminator/1
  Constant/1 -> dig_inout_tp1/1(data_in_i)
  diotp1_02_dir/1 -> dig_inout_tp1/4(direction_i)
  diotp1_02_ena/1 -> dig_inout_tp1/2(enable_i)
  diotp1_02_out/1 -> dig_inout_tp1/3(data_out_i)
  dig_inout_tp1/1(data_in_o) -> diotp1_02_in/1
  Convert7/1 -> Register7/1
  Direction/1 -> Convert7/1
  Register7/1 -> diotp1_02_dir/1
  CEP7/1 -> Register7/2
  Constant7/1 -> CEP7/1
  Convert5/1 -> Register5/1
  Enable/1 -> Convert5/1
  Register5/1 -> diotp1_02_ena/1
  CEP5/1 -> Register5/2
  Constant5/1 -> CEP5/1
  Convert3/1 -> Register3/1
  Data Out/1 -> Convert3/1
  Register3/1 -> diotp1_02_out/1
  CEP3/1 -> Register3/2
  Constant3/1 -> CEP3/1
  diotp1_02_in/1 -> Register1/1
  CEP1/1 -> Register1/2
  Constant1/1 -> CEP1/1
  Delay1/1 -> Data In/1
  Register1/1 -> Delay1/1

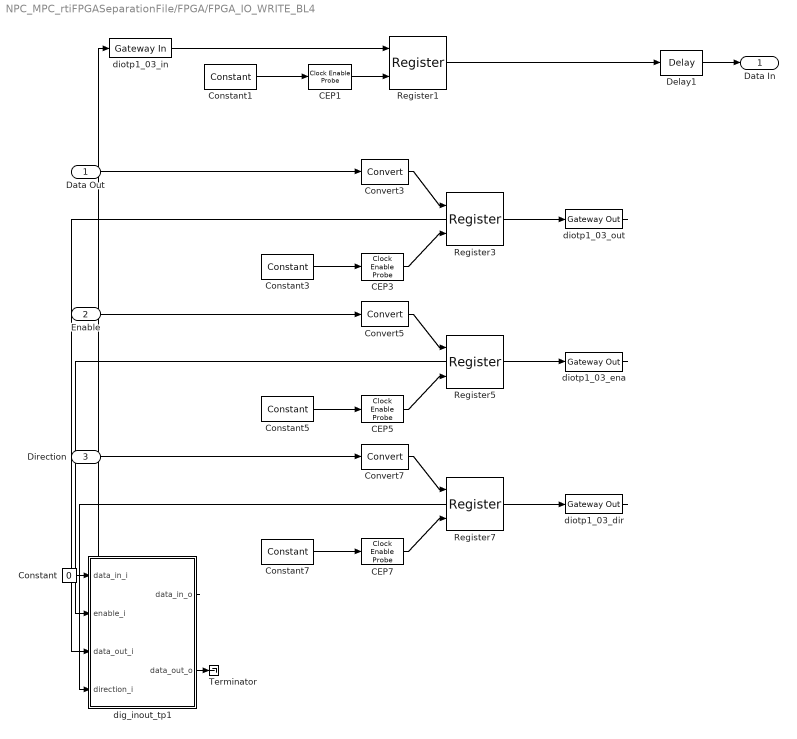
== system NPC_MPC_rtiFPGASeparationFile/FPGA/FPGA_IO_WRITE_BL4 ==
  Data Out : Inport
  Enable : Inport  Port=2
  Direction : Inport  Port=3
  CEP{1,3,5,7} (4 alike) : xbsIndex_r4/Clock Enable Probe  inherit_constraints=off  block_type=ceprobe
      settings: infoedit="Clock enable extractor.  Produces a Boolean output that mirrors the hardware clock enable associated with the input sample rate.<br><br>Hardware notes: in hardware this block costs nothing."
  Constant : Constant  Value=0
  Constant{1,3,5,7} (4 alike) : xbsIndex_r4/Constant  const=1  gui_display_data_type=Fixed-point  arith_type=Boolean  n_bits=16  bin_pt=14  preci_type=Single  exp_width=8  frac_width=24  explicit_period=on  period=1*1e-08  equ=P=C  opselect=C  inp2=PCIN>>17  opr=+  inp1=P  carry=CIN  dbl_ovrd=off  block_type=constant
  Convert3 : xbsIndex_r4/Convert  gui_display_data_type=Fixed-point  arith_type=Unsigned  n_bits=1  bin_pt=0  float_type=Single  exp_bits=8  fraction_bits=24  quantization=Truncate  overflow=Wrap  en=off  latency=0  pipeline=off  dbl_ovrd=off  block_type=convert
  Convert5 : xbsIndex_r4/Convert  gui_display_data_type=Fixed-point  arith_type=Unsigned  n_bits=1  bin_pt=0  float_type=Single  exp_bits=8  fraction_bits=24  quantization=Truncate  overflow=Wrap  en=off  latency=0  pipeline=off  dbl_ovrd=off  block_type=convert
  Convert7 : xbsIndex_r4/Convert  gui_display_data_type=Fixed-point  arith_type=Unsigned  n_bits=1  bin_pt=0  float_type=Single  exp_bits=8  fraction_bits=24  quantization=Truncate  overflow=Wrap  en=off  latency=0  pipeline=off  dbl_ovrd=off  block_type=convert
  Delay1 : xbsIndex_r4/Delay  rst=off  infoeditControl=Selection of Reset will increase slice count due to use of real FFs and instead of SRLs  en=off  latency=0  reg_retiming=off  dbl_ovrd=off  block_type=delay
  Register{1,3,5,7} (4 alike) : xbsIndex_r4/Register  init=0  rst=off  en=on  dbl_ovrd=off  block_type=register
  Terminator : Terminator
  dig_inout_tp1 : Subsystem
      mask init: same as NPC_MPC_rtiFPGASeparationFile/FPGA/FPGA_IO_WRITE_BL1/dig_inout_tp1
  diotp1_03_dir : xbsIndex_r4/Gateway Out  inherit_from_input=off  hdl_port=on  rows=1  columns=1  UseAsDAC=off  DACChannel='1'  interface=None  automatic_assignment=on  address_offset=hex2dec('00')  intf_name=''  intf_description=''  timing_constraint=None  locs_specified=off  LOCs={}  io_standard={}  block_type=gatewayout
  diotp1_03_ena : xbsIndex_r4/Gateway Out  inherit_from_input=off  hdl_port=on  rows=1  columns=1  UseAsDAC=off  DACChannel='1'  interface=None  automatic_assignment=on  address_offset=hex2dec('00')  intf_name=''  intf_description=''  timing_constraint=None  locs_specified=off  LOCs={}  io_standard={}  block_type=gatewayout
  diotp1_03_in : xbsIndex_r4/Gateway In  gui_display_data_type=Fixed-point  arith_type=Unsigned  n_bits=1  bin_pt=0  preci_type=Single  exp_width=8  frac_width=24  rows=1  columns=1  quantization="Round  (unbiased: +/- Inf)"  overflow=Saturate  period=1e-08  UseAsADC=off  ADCChannel='1'  interface=None  automatic_assignment=on  address_offset=hex2dec('00')  intf_name=''  intf_description=''  default_value=0  timing_constraint=None  locs_specified=off  LOCs={}  io_standard={}  inherit_from_input=off  hdl_port=on  dbl_ovrd=off  block_type=gatewayin
  diotp1_03_out : xbsIndex_r4/Gateway Out  inherit_from_input=off  hdl_port=on  rows=1  columns=1  UseAsDAC=off  DACChannel='1'  interface=None  automatic_assignment=on  address_offset=hex2dec('00')  intf_name=''  intf_description=''  timing_constraint=None  locs_specified=off  LOCs={}  io_standard={}  block_type=gatewayout
  Data In : Outport
  wires:
  dig_inout_tp1/2(data_out_o) -> Terminator/1
  Constant/1 -> dig_inout_tp1/1(data_in_i)
  diotp1_03_dir/1 -> dig_inout_tp1/4(direction_i)
  diotp1_03_ena/1 -> dig_inout_tp1/2(enable_i)
  diotp1_03_out/1 -> dig_inout_tp1/3(data_out_i)
  dig_inout_tp1/1(data_in_o) -> diotp1_03_in/1
  Convert7/1 -> Register7/1
  Direction/1 -> Convert7/1
  Register7/1 -> diotp1_03_dir/1
  CEP7/1 -> Register7/2
  Constant7/1 -> CEP7/1
  Convert5/1 -> Register5/1
  Enable/1 -> Convert5/1
  Register5/1 -> diotp1_03_ena/1
  CEP5/1 -> Register5/2
  Constant5/1 -> CEP5/1
  Convert3/1 -> Register3/1
  Data Out/1 -> Convert3/1
  Register3/1 -> diotp1_03_out/1
  CEP3/1 -> Register3/2
  Constant3/1 -> CEP3/1
  diotp1_03_in/1 -> Register1/1
  CEP1/1 -> Register1/2
  Constant1/1 -> CEP1/1
  Delay1/1 -> Data In/1
  Register1/1 -> Delay1/1

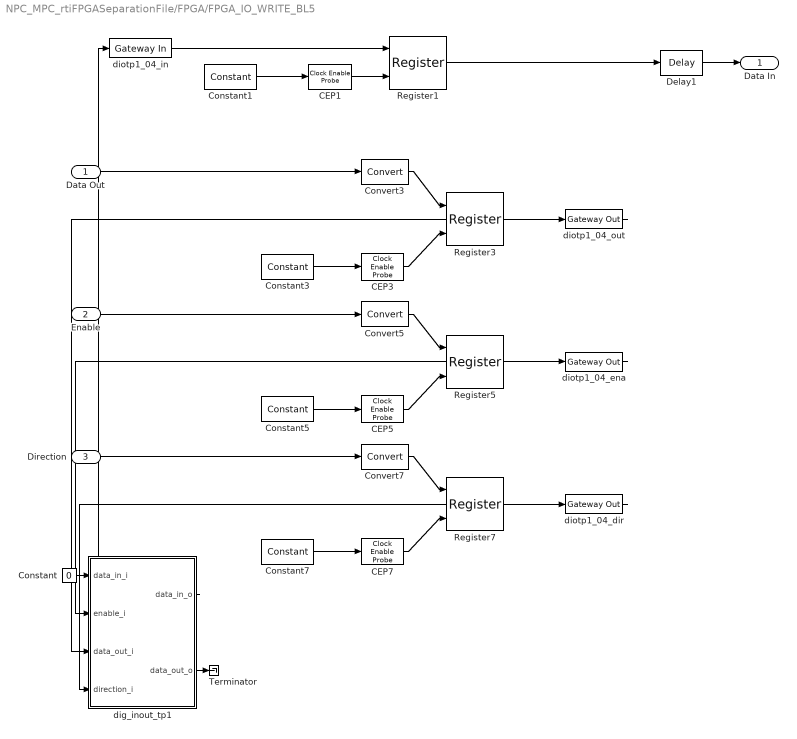
== system NPC_MPC_rtiFPGASeparationFile/FPGA/FPGA_IO_WRITE_BL5 ==
  Data Out : Inport
  Enable : Inport  Port=2
  Direction : Inport  Port=3
  CEP{1,3,5,7} (4 alike) : xbsIndex_r4/Clock Enable Probe  inherit_constraints=off  block_type=ceprobe
      settings: infoedit="Clock enable extractor.  Produces a Boolean output that mirrors the hardware clock enable associated with the input sample rate.<br><br>Hardware notes: in hardware this block costs nothing."
  Constant : Constant  Value=0
  Constant{1,3,5,7} (4 alike) : xbsIndex_r4/Constant  const=1  gui_display_data_type=Fixed-point  arith_type=Boolean  n_bits=16  bin_pt=14  preci_type=Single  exp_width=8  frac_width=24  explicit_period=on  period=1*1e-08  equ=P=C  opselect=C  inp2=PCIN>>17  opr=+  inp1=P  carry=CIN  dbl_ovrd=off  block_type=constant
  Convert3 : xbsIndex_r4/Convert  gui_display_data_type=Fixed-point  arith_type=Unsigned  n_bits=1  bin_pt=0  float_type=Single  exp_bits=8  fraction_bits=24  quantization=Truncate  overflow=Wrap  en=off  latency=0  pipeline=off  dbl_ovrd=off  block_type=convert
  Convert5 : xbsIndex_r4/Convert  gui_display_data_type=Fixed-point  arith_type=Unsigned  n_bits=1  bin_pt=0  float_type=Single  exp_bits=8  fraction_bits=24  quantization=Truncate  overflow=Wrap  en=off  latency=0  pipeline=off  dbl_ovrd=off  block_type=convert
  Convert7 : xbsIndex_r4/Convert  gui_display_data_type=Fixed-point  arith_type=Unsigned  n_bits=1  bin_pt=0  float_type=Single  exp_bits=8  fraction_bits=24  quantization=Truncate  overflow=Wrap  en=off  latency=0  pipeline=off  dbl_ovrd=off  block_type=convert
  Delay1 : xbsIndex_r4/Delay  rst=off  infoeditControl=Selection of Reset will increase slice count due to use of real FFs and instead of SRLs  en=off  latency=0  reg_retiming=off  dbl_ovrd=off  block_type=delay
  Register{1,3,5,7} (4 alike) : xbsIndex_r4/Register  init=0  rst=off  en=on  dbl_ovrd=off  block_type=register
  Terminator : Terminator
  dig_inout_tp1 : Subsystem
      mask init: same as NPC_MPC_rtiFPGASeparationFile/FPGA/FPGA_IO_WRITE_BL1/dig_inout_tp1
  diotp1_04_dir : xbsIndex_r4/Gateway Out  inherit_from_input=off  hdl_port=on  rows=1  columns=1  UseAsDAC=off  DACChannel='1'  interface=None  automatic_assignment=on  address_offset=hex2dec('00')  intf_name=''  intf_description=''  timing_constraint=None  locs_specified=off  LOCs={}  io_standard={}  block_type=gatewayout
  diotp1_04_ena : xbsIndex_r4/Gateway Out  inherit_from_input=off  hdl_port=on  rows=1  columns=1  UseAsDAC=off  DACChannel='1'  interface=None  automatic_assignment=on  address_offset=hex2dec('00')  intf_name=''  intf_description=''  timing_constraint=None  locs_specified=off  LOCs={}  io_standard={}  block_type=gatewayout
  diotp1_04_in : xbsIndex_r4/Gateway In  gui_display_data_type=Fixed-point  arith_type=Unsigned  n_bits=1  bin_pt=0  preci_type=Single  exp_width=8  frac_width=24  rows=1  columns=1  quantization="Round  (unbiased: +/- Inf)"  overflow=Saturate  period=1e-08  UseAsADC=off  ADCChannel='1'  interface=None  automatic_assignment=on  address_offset=hex2dec('00')  intf_name=''  intf_description=''  default_value=0  timing_constraint=None  locs_specified=off  LOCs={}  io_standard={}  inherit_from_input=off  hdl_port=on  dbl_ovrd=off  block_type=gatewayin
  diotp1_04_out : xbsIndex_r4/Gateway Out  inherit_from_input=off  hdl_port=on  rows=1  columns=1  UseAsDAC=off  DACChannel='1'  interface=None  automatic_assignment=on  address_offset=hex2dec('00')  intf_name=''  intf_description=''  timing_constraint=None  locs_specified=off  LOCs={}  io_standard={}  block_type=gatewayout
  Data In : Outport
  wires:
  dig_inout_tp1/2(data_out_o) -> Terminator/1
  Constant/1 -> dig_inout_tp1/1(data_in_i)
  diotp1_04_dir/1 -> dig_inout_tp1/4(direction_i)
  diotp1_04_ena/1 -> dig_inout_tp1/2(enable_i)
  diotp1_04_out/1 -> dig_inout_tp1/3(data_out_i)
  dig_inout_tp1/1(data_in_o) -> diotp1_04_in/1
  Convert7/1 -> Register7/1
  Direction/1 -> Convert7/1
  Register7/1 -> diotp1_04_dir/1
  CEP7/1 -> Register7/2
  Constant7/1 -> CEP7/1
  Convert5/1 -> Register5/1
  Enable/1 -> Convert5/1
  Register5/1 -> diotp1_04_ena/1
  CEP5/1 -> Register5/2
  Constant5/1 -> CEP5/1
  Convert3/1 -> Register3/1
  Data Out/1 -> Convert3/1
  Register3/1 -> diotp1_04_out/1
  CEP3/1 -> Register3/2
  Constant3/1 -> CEP3/1
  diotp1_04_in/1 -> Register1/1
  CEP1/1 -> Register1/2
  Constant1/1 -> CEP1/1
  Delay1/1 -> Data In/1
  Register1/1 -> Delay1/1

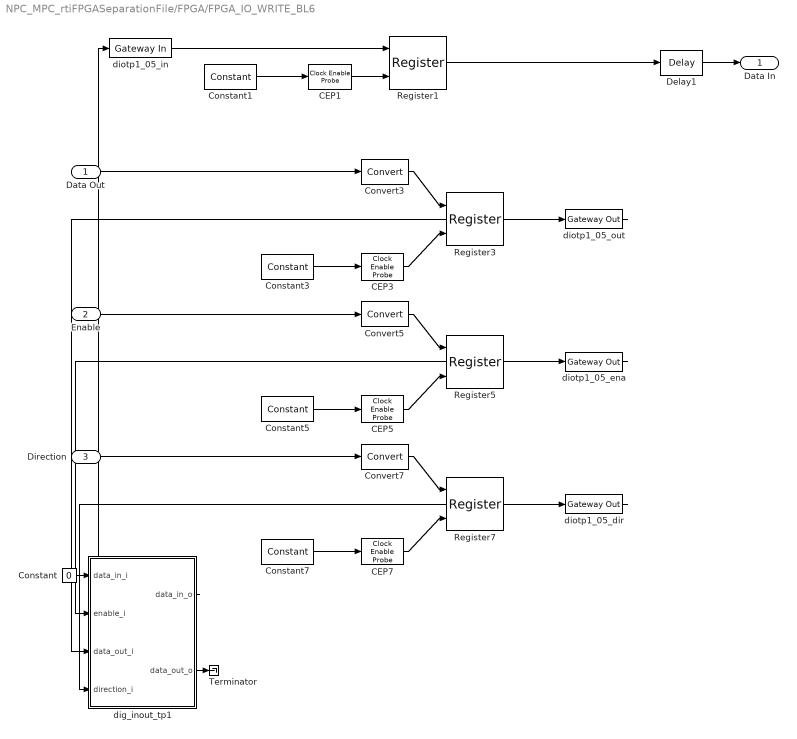
== system NPC_MPC_rtiFPGASeparationFile/FPGA/FPGA_IO_WRITE_BL6 ==
  Data Out : Inport
  Enable : Inport  Port=2
  Direction : Inport  Port=3
  CEP{1,3,5,7} (4 alike) : xbsIndex_r4/Clock Enable Probe  inherit_constraints=off  block_type=ceprobe
      settings: infoedit="Clock enable extractor.  Produces a Boolean output that mirrors the hardware clock enable associated with the input sample rate.<br><br>Hardware notes: in hardware this block costs nothing."
  Constant : Constant  Value=0
  Constant{1,3,5,7} (4 alike) : xbsIndex_r4/Constant  const=1  gui_display_data_type=Fixed-point  arith_type=Boolean  n_bits=16  bin_pt=14  preci_type=Single  exp_width=8  frac_width=24  explicit_period=on  period=1*1e-08  equ=P=C  opselect=C  inp2=PCIN>>17  opr=+  inp1=P  carry=CIN  dbl_ovrd=off  block_type=constant
  Convert3 : xbsIndex_r4/Convert  gui_display_data_type=Fixed-point  arith_type=Unsigned  n_bits=1  bin_pt=0  float_type=Single  exp_bits=8  fraction_bits=24  quantization=Truncate  overflow=Wrap  en=off  latency=0  pipeline=off  dbl_ovrd=off  block_type=convert
  Convert5 : xbsIndex_r4/Convert  gui_display_data_type=Fixed-point  arith_type=Unsigned  n_bits=1  bin_pt=0  float_type=Single  exp_bits=8  fraction_bits=24  quantization=Truncate  overflow=Wrap  en=off  latency=0  pipeline=off  dbl_ovrd=off  block_type=convert
  Convert7 : xbsIndex_r4/Convert  gui_display_data_type=Fixed-point  arith_type=Unsigned  n_bits=1  bin_pt=0  float_type=Single  exp_bits=8  fraction_bits=24  quantization=Truncate  overflow=Wrap  en=off  latency=0  pipeline=off  dbl_ovrd=off  block_type=convert
  Delay1 : xbsIndex_r4/Delay  rst=off  infoeditControl=Selection of Reset will increase slice count due to use of real FFs and instead of SRLs  en=off  latency=0  reg_retiming=off  dbl_ovrd=off  block_type=delay
  Register{1,3,5,7} (4 alike) : xbsIndex_r4/Register  init=0  rst=off  en=on  dbl_ovrd=off  block_type=register
  Terminator : Terminator
  dig_inout_tp1 : Subsystem
      mask init: same as NPC_MPC_rtiFPGASeparationFile/FPGA/FPGA_IO_WRITE_BL1/dig_inout_tp1
  diotp1_05_dir : xbsIndex_r4/Gateway Out  inherit_from_input=off  hdl_port=on  rows=1  columns=1  UseAsDAC=off  DACChannel='1'  interface=None  automatic_assignment=on  address_offset=hex2dec('00')  intf_name=''  intf_description=''  timing_constraint=None  locs_specified=off  LOCs={}  io_standard={}  block_type=gatewayout
  diotp1_05_ena : xbsIndex_r4/Gateway Out  inherit_from_input=off  hdl_port=on  rows=1  columns=1  UseAsDAC=off  DACChannel='1'  interface=None  automatic_assignment=on  address_offset=hex2dec('00')  intf_name=''  intf_description=''  timing_constraint=None  locs_specified=off  LOCs={}  io_standard={}  block_type=gatewayout
  diotp1_05_in : xbsIndex_r4/Gateway In  gui_display_data_type=Fixed-point  arith_type=Unsigned  n_bits=1  bin_pt=0  preci_type=Single  exp_width=8  frac_width=24  rows=1  columns=1  quantization="Round  (unbiased: +/- Inf)"  overflow=Saturate  period=1e-08  UseAsADC=off  ADCChannel='1'  interface=None  automatic_assignment=on  address_offset=hex2dec('00')  intf_name=''  intf_description=''  default_value=0  timing_constraint=None  locs_specified=off  LOCs={}  io_standard={}  inherit_from_input=off  hdl_port=on  dbl_ovrd=off  block_type=gatewayin
  diotp1_05_out : xbsIndex_r4/Gateway Out  inherit_from_input=off  hdl_port=on  rows=1  columns=1  UseAsDAC=off  DACChannel='1'  interface=None  automatic_assignment=on  address_offset=hex2dec('00')  intf_name=''  intf_description=''  timing_constraint=None  locs_specified=off  LOCs={}  io_standard={}  block_type=gatewayout
  Data In : Outport
  wires:
  dig_inout_tp1/2(data_out_o) -> Terminator/1
  Constant/1 -> dig_inout_tp1/1(data_in_i)
  diotp1_05_dir/1 -> dig_inout_tp1/4(direction_i)
  diotp1_05_ena/1 -> dig_inout_tp1/2(enable_i)
  diotp1_05_out/1 -> dig_inout_tp1/3(data_out_i)
  dig_inout_tp1/1(data_in_o) -> diotp1_05_in/1
  Convert7/1 -> Register7/1
  Direction/1 -> Convert7/1
  Register7/1 -> diotp1_05_dir/1
  CEP7/1 -> Register7/2
  Constant7/1 -> CEP7/1
  Convert5/1 -> Register5/1
  Enable/1 -> Convert5/1
  Register5/1 -> diotp1_05_ena/1
  CEP5/1 -> Register5/2
  Constant5/1 -> CEP5/1
  Convert3/1 -> Register3/1
  Data Out/1 -> Convert3/1
  Register3/1 -> diotp1_05_out/1
  CEP3/1 -> Register3/2
  Constant3/1 -> CEP3/1
  diotp1_05_in/1 -> Register1/1
  CEP1/1 -> Register1/2
  Constant1/1 -> CEP1/1
  Delay1/1 -> Data In/1
  Register1/1 -> Delay1/1
